simulink model "PMLSMDrive"  (R2024a)
settings: Solver=ode23t  StartTime=0.0  StopTime=10  RelTol=1e-3  AbsTol=1e-3  EnableMultiTasking=on
PreLoadFcn:
  | PMLSMDriveData;
values from neighbouring files (symbols this model uses):
  finalspeed = 0    [PMLSMDriveData.m]
  Fmax = 2000    [PMLSMDriveData.m]
  Ki_p = 100    [PMLSMDriveData.m]
  Ki_v = 250    [PMLSMDriveData.m]
  Kp_p = 200    [PMLSMDriveData.m]
  Kp_v = 250    [PMLSMDriveData.m]
  Ld = 0.01    [PMLSMDriveData.m]
  Lq = 0.01    [PMLSMDriveData.m]
  Np = pi/pitch    (= 31.4159265359)    [PMLSMDriveData.m]
  PM = 0.65    [PMLSMDriveData.m]
  Ts = 5e-5    (= 5e-05)    [PMLSMDriveData.m]
  Tsc = 1e-3    (= 0.001)    [PMLSMDriveData.m]
libraries: nesl_utility x12, fl_lib x7, ee_lib x5, eeTransforms x2, slpidlib x2, simulink x2, eePmsmCurrentController x1, eePwmGeneratorTwoLevel x1, dspsnks4 x1
CloseFcn:
  | try,close(h1_PMLSMDrive),end
  | clear h1_PMLSMDrive
  | 
  | clear PM Ld Lq L0 Rs mass pitch Np
  | clear Ts fsw Tsc Kp_id Ki_id Kp_iq Ki_iq
  | clear Kp_v Ki_v Kp_p Ki_p
Description:
  | Three-Phase PMLSM Drive
settings Model: Creator=The MathWorks, Inc.  LastModifiedBy=bkpou
settings SolverCC: AutoScaleAbsTol=off  MaxConsecutiveMinStep=2  ZeroCrossAlgorithm=Adaptive  AlgebraicLoopSolver=TrustRegion  MaxZcPerStep=1
settings DataIOCC: LimitDataPoints=on  MaxDataPoints=690000  SaveFormat=Array  ReturnWorkspaceOutputs=off  SignalLoggingName=logsout_PMLSMDrive
settings OptimizationCC: ReuseModelBlockBuffer=off  LifeSpan=inf
settings DebuggingCC: MaxConsecutiveZCsMsg=none  IgnoredZcDiagnostic=none  UnconnectedInputMsg=warning  UnconnectedOutputMsg=warning  UnconnectedLineMsg=warning  AllowSymbolicDim=off  PregeneratedLibrarySubsystemCodeDiagnostic=none  SFUnexpectedBacktrackingDiag=warning  SFNoUnconditionalDefaultTransitionDiag=warning  SFExecutionAtInitializationDiag=none  ArithmeticOperatorsInVariantConditions=warning
settings HardwareCC: ProdBitPerPointer=32  ProdBitPerSizeT=32  ProdBitPerPtrDiffT=32  ProdLargestAtomicFloat=None  ProdIntDivRoundTo=Undefined  ProdEndianess=Unspecified  ProdWordSize=32  ProdHWDeviceType=32-bit Generic
settings ModelReferenceCC: EnableRefExpFcnMdlSchedulingChecks=on  PropagateSignalLabelsOutOfModel=off
settings SFSimCC: SimUseLocalCustomCode=off
settings RTWCC: RTWUseLocalCustomCode=off  GPUComputeCapability=3.5  DLArmComputeVersion=19.05
settings CodeAppCC: StateflowObjectComments=on
settings GRTTargetCC: TargetLangStandard=C89/C90 (ANSI)
settings ConfigComp: CovMetricSettings=dw  CovSaveCumulativeToWorkspaceVar=on  CovSaveSingleToWorkspaceVar=on  CovExternalEMLEnable=off  CovSFcnEnable=off
settings SimscapeCC: SimscapeLogType=all  SimscapeLogSimulationStatistics=on  SimscapeLogName=simlog_PMLSMDrive  SimscapeLogDataHistory=690000

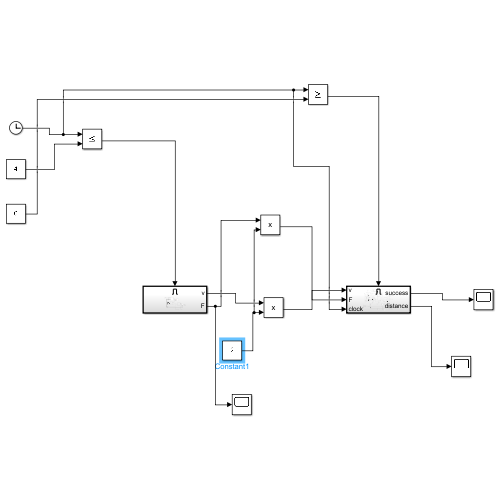
[thumbnail: Simulink's stored preview of the top-level diagram]
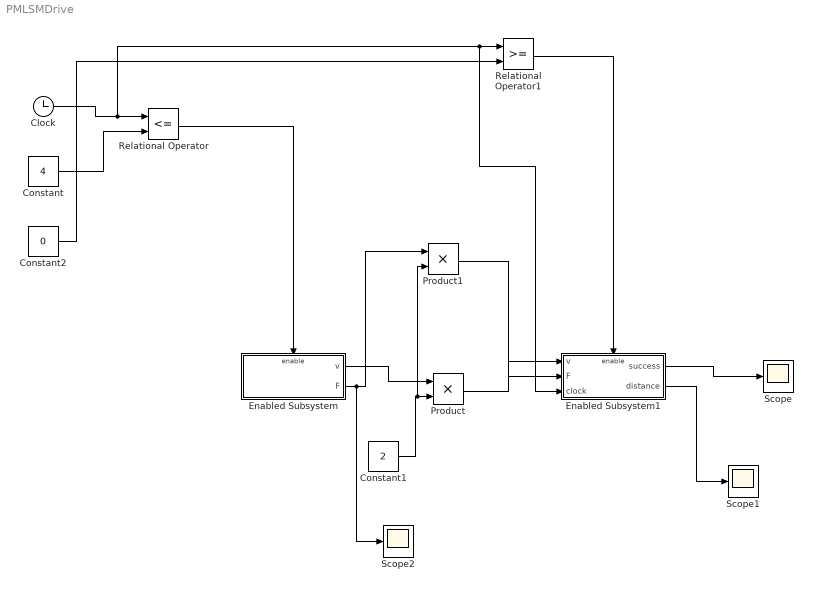
== system PMLSMDrive ==
  Clock : Clock
  Constant : Constant  Value=4
  Constant1 : Constant  Value=2
  Constant2 : Constant  Value=0
  Enabled Subsystem : Subsystem  TreatAsAtomicUnit=on
  Enabled Subsystem1 : Subsystem  TreatAsAtomicUnit=on
  Product : Product
  Product1 : Product
  Relational Operator : RelationalOperator  Operator=<=  OutDataTypeStr=boolean  RndMeth=Simplest  InputSameDT=off
  Relational Operator1 : RelationalOperator  OutDataTypeStr=boolean  RndMeth=Simplest  InputSameDT=off
  Scope : Scope
  Scope1 : Scope
  Scope2 : Scope
  wires:
  Clock/1 -> Enabled Subsystem1/3(clock), Relational Operator1/1, Relational Operator/1
  Constant/1 -> Relational Operator/2
  Relational Operator/1 -> Enabled Subsystem/Enable
  Relational Operator1/1 -> Enabled Subsystem1/Enable
  Enabled Subsystem/1(v) -> Product/1
  Constant1/1 -> Product1/2, Product/2
  Product/1 -> Enabled Subsystem1/1(v)
  Enabled Subsystem1/1(success) -> Scope/1
  Enabled Subsystem1/2(distance) -> Scope1/1
  Enabled Subsystem/2(F) -> Scope2/1, Product1/1
  Product1/1 -> Enabled Subsystem1/2(F)
  Constant2/1 -> Relational Operator1/2

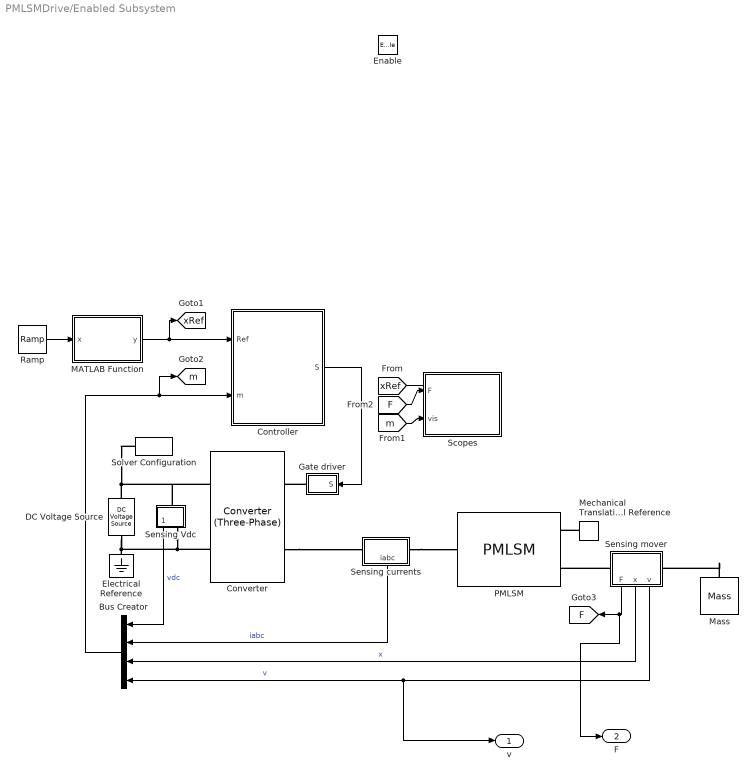
== system PMLSMDrive/Enabled Subsystem ==
  Enable : EnablePort
  Bus Creator : BusCreator  Inputs=4
  Controller : Subsystem
  Converter : ee_lib/Semiconductors & Converters/Converters/Converter (Three-Phase)  port_option=ee.enum.threePhasePort.composite  fidelity_option=ee.enum.converters.fidelity.detailed  device_type=ee.enum.converters.switchingdevice.igbt  K=0  Vf=0.8 V  Ron=0.001 Ohm  Rds=0.001 Ohm  Goff=1e-5 1/Ohm  Vgt=1 V  Vgt_off=-1 V  Ih=1 A  Vth=0.5 V  diode_param=ee.enum.converters.protectiondiode.nodynamics  diode_Vf=0.8 V  diode_Ron=0.001 Ohm  diode_Goff=1e-5 1/Ohm  diode_C=50 nF  diode_iRM=-235 A  diode_iF=300 A  diode_idot=-50 A/us  diode_trr_param=ee.enum.converters.diodetrr.trr_factor  diode_trr_factor=3  diode_trr=15 us  diode_Qrr=1.5e+3 s*uA  snubber_type=ee.enum.converters.snubber.exclude  Cs=1e-7 F  Rs=0.1 Ohm
  DC Voltage Source : ee_lib/Additional Components/SPICE Sources/DC Voltage Source  DC=220 V
  Electrical Reference : fl_lib/Electrical/Electrical Elements/Electrical Reference
  Gate driver : Subsystem
  MATLAB Function : MATLAB Function  TreatAsAtomicUnit=on
  Mass : fl_lib/Mechanical/Translational Elements/Mass  mass=mass kg  num_ports=foundation.enum.numPorts2.one  v_specify=off  v_priority=High  v=0 m/s  v_nominal_specify=off  v_nominal_value=1  v_nominal_unit=m/s  f_specify=off  f_priority=None  f=0 N  f_nominal_specify=off  f_nominal_value=1  f_nominal_unit=N
  Mechanical Translational Reference : fl_lib/Mechanical/Translational Elements/Mechanical Translational Reference
  PMLSM : ee_lib/Electromechanical/Permanent Magnet/PMLSM  port_option=ee.enum.threePhasePort.composite  winding_type=ee.enum.statorconnection.wye  machine_param=ee.enum.pmsm.parameterization.constant  polarPitch=pitch m  pmflux_param=ee.enum.pmfluxlin.fluxlinkage  pm_flux_linkage=PM Wb  force_constant=0.18 N/A  back_emf_constant=0.18 s*V/m  stator_param=ee.enum.statorparam.LdLqL0  Ld=Ld H  Lq=Lq H  idVec=[-200, 0, 200] A  iqVec=[-200, 0, 200] A  LdMatrix=0.00019 * ones(3, 3) H  LqMatrix=0.00025 * ones(3, 3) H  PmMatrix=0.03 * ones(3, 3) Wb  kfMatrix=0.18 * ones(3, 3) N/A  keMatrix=0.18 * ones(3, 3) s*V/m  L0=L0 H  Ls=0.0002 H  Lm=-0.00002 H  Ms=0.00002 H  Rs=Rs Ohm  zero_sequence=ee.enum.park.zerosequence.exclude  axes_param=ee.enum.rotorangle.qaxis  M=0 kg  lam=0 N/(m/s)  i_d_specify=on  i_d_priority=High  i_d=0 A  i_d_nominal_specify=off  i_d_nominal_value=1  i_d_nominal_unit=A  i_q_specify=on  i_q_priority=High  i_q=0 A  i_q_nominal_specify=off  i_q_nominal_value=1  i_q_nominal_unit=A  force_specify=off  force_priority=None  force=0 N  force_nominal_specify=off  force_nominal_value=1  force_nominal_unit=N  linear_velocity_specify=off  linear_velocity_priority=High  linear_velocity=0 m/s  linear_velocity_nominal_specify=off  linear_velocity_nominal_value=1  linear_velocity_nominal_unit=m/s  linear_position_specify=off  linear_position_priority=High  linear_position=0 m  linear_position_nominal_specify=off  linear_position_nominal_value=1  linear_position_nominal_unit=m  Tmeas=298.15 K  alpha=3.93e-3 1/K  alpha_flux=-0.001 1/K  stator_thermal_mass=100 J/K  rotor_thermal_mass=200 J/K  temperatureA_specify=off  temperatureA_priority=High  temperatureA=25 degC  temperatureA_nominal_specify=off  temperatureA_nominal_value=1  temperatureA_nominal_unit=degC  temperatureB_specify=off  temperatureB_priority=High  temperatureB=25 degC  temperatureB_nominal_specify=off  temperatureB_nominal_value=1  temperatureB_nominal_unit=degC  temperatureC_specify=off  temperatureC_priority=High  temperatureC=25 degC  temperatureC_nominal_specify=off  temperatureC_nominal_value=1  temperatureC_nominal_unit=degC  temperatureR_specify=off  temperatureR_priority=High  temperatureR=25 degC  temperatureR_nominal_specify=off  temperatureR_nominal_value=1  temperatureR_nominal_unit=degC
      settings: InternalSimscapePortConfiguration="{\"Bottom\":[],\"Left\":[{\"id\":\"N\",\"label\":\"~\",\"type\":\"foundation.electrical.three_phase\"}],\"Right\":[{\"id\":\"R\",\"label\":\"R\",\"type\":\"foundation.mechanical.translational.translational\"},{\"id\":\"C\",\"label\":\"C\",\"type\":\"foundation.mechanical.translational.translational\"}],\"Top\":[]}"
  Ramp : simulink/Sources/Ramp  slope=5  start=0  InitialOutput=0
  Scopes : Subsystem
  Sensing Vdc : Subsystem
      mask Display: disp('vdc')
  Sensing currents : Subsystem
      settings: PortSchema="{\"entries\":[{\"content\":{\"sides\":[{\"content\":{\"connectorIds\":[\"LConn1\"]},\"type\":\"ConnectorPlacement.EquallySpacedRectSide\",\"uuid\":\"0c76379d-baff-4140-87e0-7680e80a3e64\"},{\"content\":{\"connectorIds\":[\"RConn1\"],\"side\":\"RIGHT\"},\"type\":\"ConnectorPlacement.EquallySpacedRectSide\",\"uuid\":\"435fa78d-19d1-48b9-8f1c-afd8cf746df8\"},{\"content\":{\"connectorIds\":[],\"side\":\"TOP\"},\"type\":\"ConnectorPlacement.EquallySpacedRectSide\",\"uuid\":\"64f7027d-3f1c-43c6-9f97-24bcd914447a\"},{\"content\":{\"connectorIds\":[\"Out1\"],\"side\":\"BOTTOM\"},\"type\":\"ConnectorPlacement.EquallySpacedRectSide\",\"uuid\":\"10c10308-e912-4df5-9465-b109ad6411e6\"}]},\"type\":\"ConnectorPlacement.EquallySpacedConnector\",\"uuid\":\"559fa4aa-2e9f-4f72-acfb-6b72122ee549\"}],\"packageUris\":[\"http://schema.mathworks.com/mf0/Connector/R2020b\"],\"version\":\"1.0\"}"
      mask Display: disp('iabc')
  "Sensing mover " : Subsystem
      settings: PortSchema="{\"entries\":[{\"content\":{\"sides\":[{\"content\":{\"connectorIds\":[\"LConn1\"]},\"type\":\"ConnectorPlacement.EquallySpacedRectSide\",\"uuid\":\"6dd62e1f-51ba-4aba-a162-82178346648e\"},{\"content\":{\"connectorIds\":[\"RConn1\"],\"side\":\"RIGHT\"},\"type\":\"ConnectorPlacement.EquallySpacedRectSide\",\"uuid\":\"d7237c3a-82f8-4015-b1be-086487fff7ab\"},{\"content\":{\"connectorIds\":[],\"side\":\"TOP\"},\"type\":\"ConnectorPlacement.EquallySpacedRectSide\",\"uuid\":\"056d6889-c837-4b54-b9b7-572481429841\"},{\"content\":{\"connectorIds\":[\"Out1\",\"Out2\",\"Out3\"],\"side\":\"BOTTOM\"},\"type\":\"ConnectorPlacement.EquallySpacedRectSide\",\"uuid\":\"c892334a-0cdf-49f0-9b4f-3c9e9a0dee4e\"}]},\"type\":\"ConnectorPlacement.EquallySpacedConnector\",\"uuid\":\"04d69959-dab1-4865-ab7f-ace877df7771\"}],\"packageUris\":[\"http://schema.mathworks.com/mf0/Connector/R2020b\"],\"version\":\"1.0\"}"
  Solver Configuration : nesl_utility/Solver Configuration  PhysicalDomain=network_engine_domain  SubClassName=solver  LeftPortType=input  RightPortType=generic  Tones=[]  Harmonics=[]  SimulateNoise=off  Profile=off  UseLocalSampling=off  EnableSwitchedLinearOptims=on  FrequencyDomain=off  UseCCode=off  RelTol=0.001  AbsTol=1e-06  MinStep=1e-09  ToWorkspace=off  RevertToSquareIcSolve=off  NumHomotopyIterations=100  PhasorMode=off  PhasorModeNumHarmonics=1  ConsistencySolver=NEWTON_FTOL  IndexReductionMethod=DerivativeReplacement  DoDC=off  ResidualTolerance=1e-9  ConsistencyTolSource=GLOBAL  ConsistencyAbsTol=0.001  ConsistencyRelTol=0.001  ConsistencyTolFactor=0.001  UseLocalSolver=on  LocalSolverChoice=NE_PARTITIONING_ADVANCER  ResolveIndetEquations=on  FunctionEvalNumThread=1  LocalSolverSampleTime=Ts  DoFixedCost=on  MaxNonlinIter=4  MaxModeIter=2  ComputeImpulses=off  ImpulseIterations=2  LinearAlgebra=auto  LinearAlgebraNumThread=0  EquationFormulation=NE_TIME_EF  DelaysMemoryBudget=1024  AutomaticFiltering=on  FilteringTimeConstant=0.001  PartitionStorageMethod=AS_NEEDED  PartitionMemoryBudget=1024  PartitionMethod=ROBUST  MultibodyUseLocalSolver=off  MultibodyLocalSolverChoice=ODE1  MultibodyLocalSolverSampleTime=0.001
  v : Outport
  F : Outport  Port=2
  tag scope: F=global, m=global, xRef=global
  wires:
  Ramp/1 -> MATLAB Function/1(x)
  "Sensing mover "/2(x) -> Bus Creator/3  "x"
  Sensing currents/1(iabc) -> Bus Creator/2  "iabc"
  "Sensing mover "/3(v) -> v/1, Bus Creator/4  "v"
  Bus Creator/1 -> [m], Controller/2(m)
  [m] -> Scopes/2(vis)
  Controller/1(S) -> Gate driver/1(S)
  "Sensing mover "/1(F) -> F/1, [F]
  [F] -> Scopes/1(F)
  [xRef] -> ?
  MATLAB Function/1(y) -> [xRef], Controller/1(Ref)
  Sensing Vdc/1(vdc) -> Bus Creator/1  "vdc"
  connections:
  Converter/RConn2 -- DC Voltage Source/RConn1 -- Electrical Reference/LConn1 -- Sensing Vdc/RConn1
  Solver Configuration/RConn1 -- DC Voltage Source/LConn1 -- Sensing Vdc/LConn1 -- Converter/RConn1
  Mass/LConn1 -- "Sensing mover "/RConn1
  Gate driver/RConn1 -- Converter/LConn1
  Sensing currents/RConn1 -- PMLSM/LConn1
  "Sensing mover "/LConn1 -- PMLSM/RConn1
  Converter/LConn2 -- Sensing currents/LConn1
  Mechanical Translational Reference/LConn1 -- PMLSM/RConn2

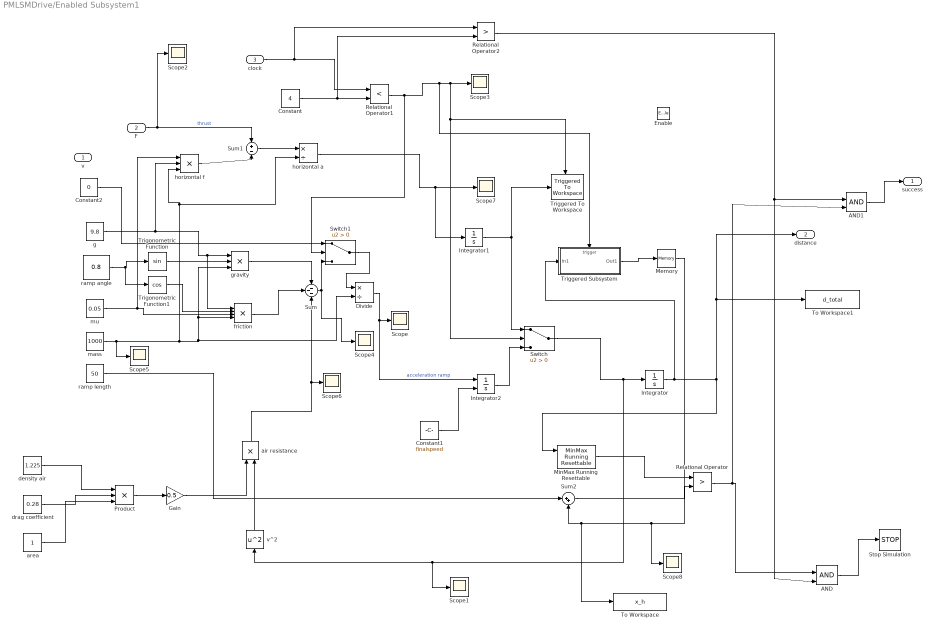
== system PMLSMDrive/Enabled Subsystem1 ==
  v : Inport
  F : Inport  Port=2
  clock : Inport  Port=3
  Enable : EnablePort
  AND : Logic  IconShape=distinctive  AllPortsSameDT=off  OutDataTypeStr=boolean
  AND1 : Logic  IconShape=distinctive  AllPortsSameDT=off  OutDataTypeStr=boolean
  Constant : Constant  Value=4
  Constant1 : Constant  Value=finalspeed
  Constant2 : Constant  Value=0
  Divide : Product  Inputs=*/
  Gain : Gain  Gain=0.5
  Integrator : Integrator
  Integrator1 : Integrator
  Integrator2 : Integrator  InitialConditionSource=external
  Memory : Memory
  MinMax Running Resettable : simulink/Math Operations/MinMax Running Resettable  Function=max  vinit=0.0
  Product : Product  Inputs=3
  Relational Operator : RelationalOperator  Operator=>  OutDataTypeStr=boolean  RndMeth=Simplest  InputSameDT=off
  Relational Operator1 : RelationalOperator  Operator=<  OutDataTypeStr=boolean  RndMeth=Simplest  InputSameDT=off
  Relational Operator2 : RelationalOperator  Operator=>  OutDataTypeStr=boolean  RndMeth=Simplest  InputSameDT=off
  Scope{,1..8} (9 alike) : Scope
  Stop Simulation : Stop
  Sum : Sum  Inputs=---
  Sum1 : Sum  Inputs=+-
  Sum2 : Sum  Inputs=|++
  Switch : Switch  Criteria=u2 > Threshold  SaturateOnIntegerOverflow=off  InputSameDT=off
  Switch1 : Switch  Criteria=u2 > Threshold  SaturateOnIntegerOverflow=off  InputSameDT=off
  To Workspace : ToWorkspace  VariableName=x_h  SaveFormat=Timeseries  SampleTime=-1
  To Workspace1 : ToWorkspace  VariableName=d_total  SaveFormat=Timeseries  SampleTime=-1
  Triggered Subsystem : Subsystem  TreatAsAtomicUnit=on
  Triggered To Workspace : dspsnks4/Triggered To Workspace  TriggerType=Falling edge  VariableName=finalspeed  Buffer=1  Save2DMode=2-D array (concatenate along first dimension)
      settings: FixptAsFi=off
  Trigonometric Function : Trigonometry
  Trigonometric Function1 : Trigonometry  Operator=cos
  air resistance : Product
  area : Constant
  density air : Constant  Value=1.225
  drag coefficient : Constant  Value=0.28
  friction : Product  Inputs=4
  g : Constant  Value=9.8
  gravity : Product  Inputs=3
  horizontal a : Product  Inputs=*/
  horizontal f : Product  Inputs=3
  mass : Constant  Value=1000
  mu : Constant  Value=0.05
  ramp angle : Constant  Value=0.8
  ramp length : Constant  Value=50
  v^2 : Math  Operator=square
  success : Outport
  distance : Outport  Port=2
  wires:
  ramp angle/1 -> Trigonometric Function1/1, Trigonometric Function/1
  mass/1 -> Scope5/1, horizontal a/2, horizontal f/3, Divide/2, friction/4, gravity/3
  g/1 -> horizontal f/2, friction/1, gravity/1
  Trigonometric Function/1 -> gravity/2
  Trigonometric Function1/1 -> friction/2
  mu/1 -> horizontal f/1, friction/3
  gravity/1 -> Sum/1
  friction/1 -> Sum/2
  Integrator/1 -> Triggered Subsystem/1(In1), MinMax Running Resettable/1, distance/1, To Workspace1/1
  MinMax Running Resettable/1 -> Relational Operator/1
  Relational Operator/1 -> AND1/2, AND/1
  density air/1 -> Product/1
  drag coefficient/1 -> Product/2
  area/1 -> Product/3
  Product/1 -> Gain/1
  Gain/1 -> air resistance/1
  air resistance/1 -> Scope6/1, Sum/3
  v^2/1 -> air resistance/2
  F/1 -> Sum1/1, Scope2/1  "thrust"
  horizontal f/1 -> Sum1/2
  Sum1/1 -> horizontal a/1
  horizontal a/1 -> Integrator1/1, Scope7/1
  Relational Operator1/1 -> Switch1/2, Triggered Subsystem/Trigger, Triggered To Workspace/Trigger, Switch/2, Scope3/1
  Integrator1/1 -> Switch/1, Triggered To Workspace/1
  Switch/1 -> Scope1/1, v^2/1, Integrator/1
  Integrator2/1 -> Switch/3
  Divide/1 -> Scope/1, Integrator2/1  "acceleration ramp"
  Switch1/1 -> Divide/1
  Constant2/1 -> Switch1/1
  Sum/1 -> Switch1/3, Scope4/1
  Constant/1 -> Relational Operator2/2, Relational Operator1/2
  clock/1 -> Relational Operator2/1, Relational Operator1/1
  Constant1/1 -> Integrator2/2
  ramp length/1 -> Sum2/1
  Sum2/1 -> Relational Operator/2
  Triggered Subsystem/1(Out1) -> Memory/1
  Memory/1 -> Scope8/1, To Workspace/1, Sum2/2
  Relational Operator2/1 -> AND1/1, AND/2
  AND/1 -> Stop Simulation/1
  AND1/1 -> success/1

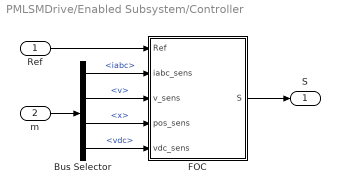
== system PMLSMDrive/Enabled Subsystem/Controller ==
  Ref : Inport
  m : Inport  Port=2
  Bus Selector : BusSelector  OutputSignals=iabc,v,x,vdc
  FOC : Subsystem
  S : Outport
  wires:
  Bus Selector/2 -> FOC/3(v_sens)  "<v>"
  Bus Selector/4 -> FOC/5(vdc_sens)  "<vdc>"
  Bus Selector/3 -> FOC/4(pos_sens)  "<x>"
  Bus Selector/1 -> FOC/2(iabc_sens)  "<iabc>"
  Ref/1 -> FOC/1(Ref)
  FOC/1(S) -> S/1
  m/1 -> Bus Selector/1

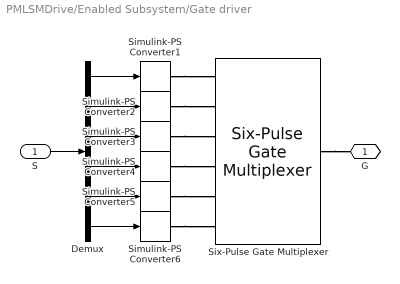
== system PMLSMDrive/Enabled Subsystem/Gate driver ==
  S : Inport
  Demux : Demux  Outputs=6
  Simulink-PS Converter{1..6} (6 alike) : nesl_utility/Simulink-PS Converter  PhysicalDomain=network_engine_domain  SubClassName=ps_input  LeftPortType=input  RightPortType=output  PseudoPeriodic=off  Frequencies=[]  NoiseDistribution=none  NoiseParameters=[]  Unit=1  AffineConversion=off  FilteringAndDerivatives=zero  SimscapeFilterOrder=1  InputFilterTimeConstant=0.001  UdotUserProvided=1
  Six-Pulse Gate Multiplexer : ee_lib/Semiconductors & Converters/Converters/Six-Pulse Gate Multiplexer  port_option=ee.enum.controlport.ps
  G : PMIOPort  Side=Right
  wires:
  Demux/1 -> Simulink-PS Converter1/1
  S/1 -> Demux/1
  Demux/4 -> Simulink-PS Converter4/1
  Demux/2 -> Simulink-PS Converter2/1
  Demux/3 -> Simulink-PS Converter3/1
  Demux/5 -> Simulink-PS Converter5/1
  Demux/6 -> Simulink-PS Converter6/1
  connections:
  Six-Pulse Gate Multiplexer/RConn1 -- G/RConn1
  Simulink-PS Converter1/RConn1 -- Six-Pulse Gate Multiplexer/LConn1
  Simulink-PS Converter3/RConn1 -- Six-Pulse Gate Multiplexer/LConn3
  Simulink-PS Converter5/RConn1 -- Six-Pulse Gate Multiplexer/LConn5
  Simulink-PS Converter6/RConn1 -- Six-Pulse Gate Multiplexer/LConn6
  Simulink-PS Converter4/RConn1 -- Six-Pulse Gate Multiplexer/LConn4
  Simulink-PS Converter2/RConn1 -- Six-Pulse Gate Multiplexer/LConn2

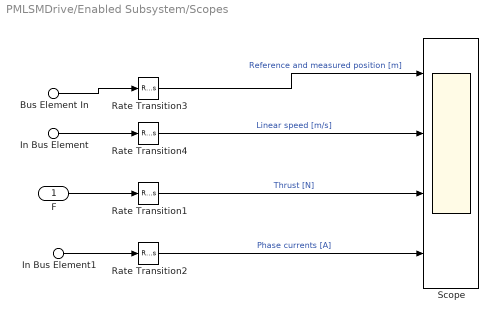
== system PMLSMDrive/Enabled Subsystem/Scopes ==
  F : Inport
  Bus Element In : Inport  Port=2  PortName=vis  Element=x
  In Bus Element : Inport  Port=2  PortName=vis  Element=v
  In Bus Element1 : Inport  Port=2  PortName=vis  Element=iabc
  Rate Transition{1..4} (4 alike) : RateTransition  OutPortSampleTime=Tsc
  Scope : Scope  NumInputPorts=4
  wires:
  In Bus Element/1 -> Rate Transition4/1
  Rate Transition2/1 -> Scope/4  "Phase currents [A]"
  In Bus Element1/1 -> Rate Transition2/1
  F/1 -> Rate Transition1/1
  Rate Transition1/1 -> Scope/3  "Thrust [N]"
  Bus Element In/1 -> Rate Transition3/1
  Rate Transition3/1 -> Scope/1  "Reference and measured position [m]"
  Rate Transition4/1 -> Scope/2  "Linear speed [m/s]"

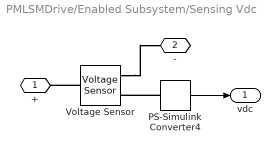
== system PMLSMDrive/Enabled Subsystem/Sensing Vdc ==
  PS-Simulink Converter4 : nesl_utility/PS-Simulink Converter  PhysicalDomain=network_engine_domain  SubClassName=ps_output  LeftPortType=input  RightPortType=output  PseudoPeriodic=off  Frequencies=[]  VectorFormat=1-D array  Unit=V  AffineConversion=off
  Voltage Sensor : fl_lib/Electrical/Electrical Sensors/Voltage Sensor
  + : PMIOPort  Side=Left
  - : PMIOPort  Port=2  Side=Right
  vdc : Outport
  wires:
  PS-Simulink Converter4/1 -> vdc/1
  connections:
  Voltage Sensor/LConn1 -- +/RConn1
  Voltage Sensor/RConn2 -- -/RConn1
  PS-Simulink Converter4/LConn1 -- Voltage Sensor/RConn1

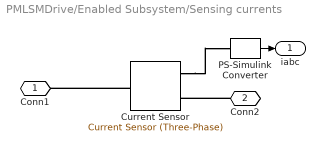
== system PMLSMDrive/Enabled Subsystem/Sensing currents ==
  Current Sensor : ee_lib/Sensors & Transducers/Current Sensor (Three-Phase)
  PS-Simulink Converter : nesl_utility/PS-Simulink Converter  PhysicalDomain=network_engine_domain  SubClassName=ps_output  LeftPortType=input  RightPortType=output  PseudoPeriodic=off  Frequencies=[]  VectorFormat=1-D array  Unit=A  AffineConversion=off
  Conn1 : PMIOPort  Side=Left
  Conn2 : PMIOPort  Port=2  Side=Right
  iabc : Outport
  wires:
  PS-Simulink Converter/1 -> iabc/1
  connections:
  Current Sensor/RConn1 -- PS-Simulink Converter/LConn1
  Conn2/RConn1 -- Current Sensor/RConn2
  Current Sensor/LConn1 -- Conn1/RConn1

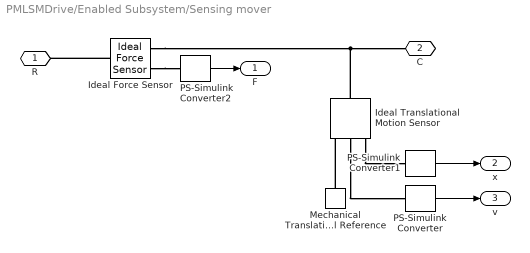
== system PMLSMDrive/Enabled Subsystem/Sensing mover  ==
  Ideal Force Sensor : fl_lib/Mechanical/Mechanical Sensors/Ideal Force Sensor
  Ideal Translational Motion Sensor : fl_lib/Mechanical/Mechanical Sensors/Ideal Translational Motion Sensor  reference=foundation.enum.MeasurementReference.difference  acceleration_port=false  velocity_port=true  position_port=true  offset=0 m
  Mechanical Translational Reference : fl_lib/Mechanical/Translational Elements/Mechanical Translational Reference
  PS-Simulink Converter : nesl_utility/PS-Simulink Converter  PhysicalDomain=network_engine_domain  SubClassName=ps_output  LeftPortType=input  RightPortType=output  PseudoPeriodic=off  Frequencies=[]  VectorFormat=1-D array  Unit=m/s  AffineConversion=off
  PS-Simulink Converter1 : nesl_utility/PS-Simulink Converter  PhysicalDomain=network_engine_domain  SubClassName=ps_output  LeftPortType=input  RightPortType=output  PseudoPeriodic=off  Frequencies=[]  VectorFormat=1-D array  Unit=m  AffineConversion=off
  PS-Simulink Converter2 : nesl_utility/PS-Simulink Converter  PhysicalDomain=network_engine_domain  SubClassName=ps_output  LeftPortType=input  RightPortType=output  PseudoPeriodic=off  Frequencies=[]  VectorFormat=1-D array  Unit=N  AffineConversion=off
  R : PMIOPort  Side=Left
  C : PMIOPort  Port=2  Side=Right
  F : Outport
  x : Outport  Port=2
  v : Outport  Port=3
  wires:
  PS-Simulink Converter2/1 -> F/1
  PS-Simulink Converter/1 -> v/1
  PS-Simulink Converter1/1 -> x/1
  connections:
  Ideal Force Sensor/LConn1 -- R/RConn1
  Ideal Force Sensor/RConn2 -- PS-Simulink Converter2/LConn1
  Ideal Force Sensor/RConn1 -- Ideal Translational Motion Sensor/LConn1 -- C/RConn1
  Ideal Translational Motion Sensor/RConn3 -- PS-Simulink Converter1/LConn1
  Ideal Translational Motion Sensor/RConn2 -- PS-Simulink Converter/LConn1
  Mechanical Translational Reference/LConn1 -- Ideal Translational Motion Sensor/RConn1

== system PMLSMDrive/Enabled Subsystem1/Triggered Subsystem ==
  In1 : Inport
  Trigger : TriggerPort  TriggerType=falling  VariantControl=(inherit)
  Out1 : Outport
  wires:
  In1/1 -> Out1/1

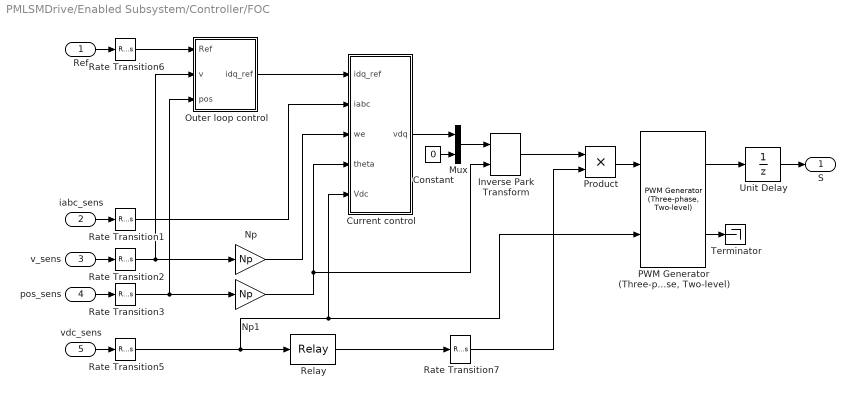
== system PMLSMDrive/Enabled Subsystem/Controller/FOC ==
  Ref : Inport
  iabc_sens : Inport  Port=2
  v_sens : Inport  Port=3
  pos_sens : Inport  Port=4
  vdc_sens : Inport  Port=5
  Constant : Constant  Value=0  SampleTime=-1
  Current control : Subsystem
  Inverse Park Transform : eeTransforms/Inverse Park Transform  AxisAlignment=Q-axis  PowerInvariant=off
  Mux : Mux  Inputs=2
  Np : Gain  Gain=Np
  Np1 : Gain  Gain=Np
  Outer loop control : Subsystem
  "PWM Generator (Three-phase, Two-level)" : eePwmGeneratorTwoLevel/PWM Generator (Three-phase, Two-level)  PWMMode=Continuous PWM (CPWM)  CPWMMode=SVM: space vector modulation  DPWMMode=60 DPWM: 60 degree discontinuous PWM  fsw=fsw  Ts=Ts
  Product : Product
  Rate Transition{1..3,5..6} (5 alike) : RateTransition  OutPortSampleTime=Tsc
  Rate Transition7 : RateTransition  OutPortSampleTime=Ts
  Relay : Relay  OnSwitchValue=24  OffSwitchValue=12
  Terminator : Terminator
  Unit Delay : UnitDelay  SampleTime=Ts  HasFrameUpgradeWarning=on
  S : Outport  VectorParamsAs1DForOutWhenUnconnected=off
  wires:
  v_sens/1 -> Rate Transition2/1
  pos_sens/1 -> Rate Transition3/1
  Current control/1(vdq) -> Mux/1
  Mux/1 -> Inverse Park Transform/1
  Rate Transition1/1 -> Current control/2(iabc)
  Outer loop control/1(idq_ref) -> Current control/1(idq_ref)
  Rate Transition5/1 -> Relay/1, "PWM Generator (Three-phase, Two-level)"/2, Current control/5(Vdc)
  vdc_sens/1 -> Rate Transition5/1
  iabc_sens/1 -> Rate Transition1/1
  Rate Transition3/1 -> Np1/1, Outer loop control/3(pos)
  Constant/1 -> Mux/2
  Relay/1 -> Rate Transition7/1
  Rate Transition2/1 -> Np/1, Outer loop control/2(v)
  Ref/1 -> Rate Transition6/1
  "PWM Generator (Three-phase, Two-level)"/2 -> Terminator/1
  Unit Delay/1 -> S/1
  Np/1 -> Current control/3(we)
  Np1/1 -> Current control/4(theta), Inverse Park Transform/2
  Rate Transition6/1 -> Outer loop control/1(Ref)
  "PWM Generator (Three-phase, Two-level)"/1 -> Unit Delay/1
  Product/1 -> "PWM Generator (Three-phase, Two-level)"/1
  Inverse Park Transform/1 -> Product/1
  Rate Transition7/1 -> Product/2

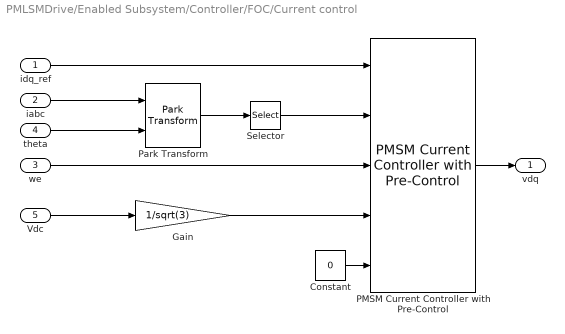
== system PMLSMDrive/Enabled Subsystem/Controller/FOC/Current control ==
  idq_ref : Inport
  iabc : Inport  Port=2
  we : Inport  Port=3
  theta : Inport  Port=4
  Vdc : Inport  Port=5
  Constant : Constant  Value=0  SampleTime=-1
  Gain : Gain  Gain=1/sqrt(3)
  PMSM Current Controller with Pre-Control : eePmsmCurrentController/PMSM Current Controller with Pre-Control  Kp_id=Kp_id  Ki_id=Ki_id  Kaw_id=1  Kp_iq=Kp_iq  Ki_iq=Ki_iq  Kaw_iq=1  Ts=-1  Tsd=Tsc  AxisPrio=Q-axis  ActZC=on  ActFF=on  idVect=[-200, 0, 200]  iqVect=[-200, 0, 200]  LdMatrix=Ld * ones(3, 3)  LqMatrix=Lq * ones(3, 3)  psimMatrix=PM * ones(3, 3)
  Park Transform : eeTransforms/Park Transform  AxisAlignment=Q-axis  PowerInvariant=off
  Selector : Selector  InputPortWidth=3  IndexOptions=Index vector (dialog)  Indices=[1 2]  OutputSizes=1
  vdq : Outport  VectorParamsAs1DForOutWhenUnconnected=off
  wires:
  Vdc/1 -> Gain/1
  iabc/1 -> Park Transform/1
  we/1 -> PMSM Current Controller with Pre-Control/3
  theta/1 -> Park Transform/2
  PMSM Current Controller with Pre-Control/1 -> vdq/1
  idq_ref/1 -> PMSM Current Controller with Pre-Control/1
  Constant/1 -> PMSM Current Controller with Pre-Control/5
  Selector/1 -> PMSM Current Controller with Pre-Control/2
  Gain/1 -> PMSM Current Controller with Pre-Control/4
  Park Transform/1 -> Selector/1

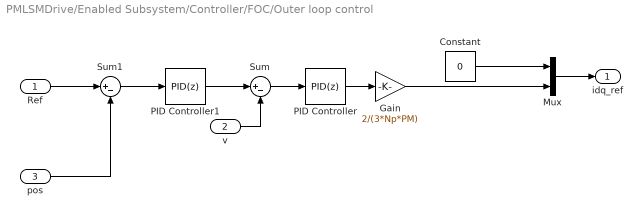
== system PMLSMDrive/Enabled Subsystem/Controller/FOC/Outer loop control ==
  Ref : Inport
  v : Inport  Port=2
  pos : Inport  Port=3
  Constant : Constant  Value=0
  Gain : Gain  Gain=2/(3*Np*PM)
  Mux : Mux  Inputs=2
  PID Controller : slpidlib/PID Controller  Controller=PID  Form=Parallel  TimeDomain=Discrete-time  UseExternalTs=off  SampleTime=Tsc  IntegratorMethod=Forward Euler  FilterMethod=Forward Euler  ControllerParametersSource=internal  P=Kp_v  I=Ki_v  UseKiTs=off  D=0  UseExternalDerivativeSource=off  N=100  UseFilter=on  TunerSelectOption=Transfer Function Based (PID Tuner App)  InitialConditionSource=internal  InitialConditionForIntegrator=0  InitialConditionForFilter=0  DifferentiatorICPrevScaledInput=0  ExternalReset=none  TrackingMode=off  Kt=1  LimitOutput=on  SatLimitsSource=internal  UpperSaturationLimit=Fmax*1.5  LowerSaturationLimit=-Fmax*1.5  LinearizeAsGain=on  AntiWindupMode=back-calculation  Kb=1000  LimitIntegrator=off  UpperIntegratorSaturationLimit=inf  LowerIntegratorSaturationLimit=-inf  POutMin=[]  POutMax=[]  IOutMin=[]  IOutMax=[]  DOutMin=[]  DOutMax=[]  NOutMin=[]  NOutMax=[]  SumOutMin=[]  SumOutMax=[]  SaturationOutMin=[]  SaturationOutMax=[]  PParamMin=[]  PParamMax=[]  IParamMin=[]  IParamMax=[]  DParamMin=[]  DParamMax=[]  NParamMin=[]  NParamMax=[]  KbParamMin=[]  KbParamMax=[]  KtParamMin=[]  KtParamMax=[]  KbOutMin=[]  KbOutMax=[]  KtOutMin=[]  KtOutMax=[]  IntegratorOutMin=[]  IntegratorOutMax=[]  FilterOutMin=[]  FilterOutMax=[]  SumI1OutMin=[]  SumI1OutMax=[]  SumI2OutMin=[]  SumI2OutMax=[]  SumI3OutMin=[]  SumI3OutMax=[]  SumI4OutMin=[]  SumI4OutMax=[]  SumDOutMin=[]  SumDOutMax=[]  DifferentiatorOutMin=[]  DifferentiatorOutMax=[]  FilterDiffOutCoefMin=[]  FilterDiffOutCoefMax=[]  ReciprocalOutMin=[]  ReciprocalOutMax=[]  SumDenOutMin=[]  SumDenOutMax=[]  SumNumOutMin=[]  SumNumOutMax=[]  DivideOutMin=[]  DivideOutMax=[]  UdiffTsProdOutMin=[]  UdiffTsProdOutMax=[]  NTsProdOutMin=[]  NTsProdOutMax=[]  UintegralTsProdOutMin=[]  UintegralTsProdOutMax=[]  UngainTsProdOutMin=[]  UngainTsProdOutMax=[]  ClampingZeroOutDataTypeStr=Inherit: Inherit via back propagation  ClampingZeroOutMin=[]  ClampingZeroOutMax=[]  FilterDenConstantOutDataTypeStr=Inherit: Inherit via back propagation  FilterDenConstantOutMin=[]  FilterDenConstantOutMax=[]  PCopyOutDataTypeStr=Inherit: Inherit via back propagation  PCopyOutMin=[]  PCopyOutMax=[]  NCopyOutDataTypeStr=Inherit: Inherit via back propagation  NCopyOutMin=[]  NCopyOutMax=[]  IntegratorContinuousStateAttributes=''  IntegratorStateMustResolveToSignalObject=off  IntegratorRTWStateStorageClass=Auto  FilterContinuousStateAttributes=''  FilterStateMustResolveToSignalObject=off  FilterRTWStateStorageClass=Auto  ParallelPVariant=InternalParameters  IdealPVariant=Disabled  IVariant=InternalParameters  DVariant=InternalParameters  IntegratorVariant=Discrete  SatVariant=Enabled  AWVariant=BackCalculation  PCopyVariant=Disabled  TRVariant=Disabled  FdbkBlocksVariant=Forward  IdealPFdbkVariant=Disabled  SatFdbkVariant=Disabled  DerivativeFilterVariant=ForwardEulerFilter  NVariant=InternalParameters  NCopyVariant=Disabled  FilterICVariant=InternalICsFilter  IntegratorICVariant=InternalICs  ExternalResetVariant=Disabled  TRSumVariant=Passthrough  SumFdbkVariant=Disabled  SumVariant=Sum_PID  TsampFilterVariant=InternalTs  TsampNgainVariant=Passthrough  TsampIntegralVariant=Disabled_SignalSpec  ExternalSaturationOutDataTypeStr=Inherit: Same as second input  DerivativeSourceVariant=ErrorSignal
  PID Controller1 : slpidlib/PID Controller  Controller=PID  Form=Parallel  TimeDomain=Discrete-time  UseExternalTs=off  SampleTime=Tsc  IntegratorMethod=Forward Euler  FilterMethod=Forward Euler  ControllerParametersSource=internal  P=Kp_p  I=Ki_p  UseKiTs=off  D=0  UseExternalDerivativeSource=off  N=100  UseFilter=on  TunerSelectOption=Transfer Function Based (PID Tuner App)  InitialConditionSource=internal  InitialConditionForIntegrator=0  InitialConditionForFilter=0  DifferentiatorICPrevScaledInput=0  ExternalReset=none  TrackingMode=off  Kt=1  LimitOutput=on  SatLimitsSource=internal  UpperSaturationLimit=10  LowerSaturationLimit=-10  LinearizeAsGain=on  AntiWindupMode=back-calculation  Kb=1000  LimitIntegrator=off  UpperIntegratorSaturationLimit=inf  LowerIntegratorSaturationLimit=-inf  POutMin=[]  POutMax=[]  IOutMin=[]  IOutMax=[]  DOutMin=[]  DOutMax=[]  NOutMin=[]  NOutMax=[]  SumOutMin=[]  SumOutMax=[]  SaturationOutMin=[]  SaturationOutMax=[]  PParamMin=[]  PParamMax=[]  IParamMin=[]  IParamMax=[]  DParamMin=[]  DParamMax=[]  NParamMin=[]  NParamMax=[]  KbParamMin=[]  KbParamMax=[]  KtParamMin=[]  KtParamMax=[]  KbOutMin=[]  KbOutMax=[]  KtOutMin=[]  KtOutMax=[]  IntegratorOutMin=[]  IntegratorOutMax=[]  FilterOutMin=[]  FilterOutMax=[]  SumI1OutMin=[]  SumI1OutMax=[]  SumI2OutMin=[]  SumI2OutMax=[]  SumI3OutMin=[]  SumI3OutMax=[]  SumI4OutMin=[]  SumI4OutMax=[]  SumDOutMin=[]  SumDOutMax=[]  DifferentiatorOutMin=[]  DifferentiatorOutMax=[]  FilterDiffOutCoefMin=[]  FilterDiffOutCoefMax=[]  ReciprocalOutMin=[]  ReciprocalOutMax=[]  SumDenOutMin=[]  SumDenOutMax=[]  SumNumOutMin=[]  SumNumOutMax=[]  DivideOutMin=[]  DivideOutMax=[]  UdiffTsProdOutMin=[]  UdiffTsProdOutMax=[]  NTsProdOutMin=[]  NTsProdOutMax=[]  UintegralTsProdOutMin=[]  UintegralTsProdOutMax=[]  UngainTsProdOutMin=[]  UngainTsProdOutMax=[]  ClampingZeroOutDataTypeStr=Inherit: Inherit via back propagation  ClampingZeroOutMin=[]  ClampingZeroOutMax=[]  FilterDenConstantOutDataTypeStr=Inherit: Inherit via back propagation  FilterDenConstantOutMin=[]  FilterDenConstantOutMax=[]  PCopyOutDataTypeStr=Inherit: Inherit via back propagation  PCopyOutMin=[]  PCopyOutMax=[]  NCopyOutDataTypeStr=Inherit: Inherit via back propagation  NCopyOutMin=[]  NCopyOutMax=[]  IntegratorContinuousStateAttributes=''  IntegratorStateMustResolveToSignalObject=off  IntegratorRTWStateStorageClass=Auto  FilterContinuousStateAttributes=''  FilterStateMustResolveToSignalObject=off  FilterRTWStateStorageClass=Auto  ParallelPVariant=InternalParameters  IdealPVariant=Disabled  IVariant=InternalParameters  DVariant=InternalParameters  IntegratorVariant=Discrete  SatVariant=Enabled  AWVariant=BackCalculation  PCopyVariant=Disabled  TRVariant=Disabled  FdbkBlocksVariant=Forward  IdealPFdbkVariant=Disabled  SatFdbkVariant=Disabled  DerivativeFilterVariant=ForwardEulerFilter  NVariant=InternalParameters  NCopyVariant=Disabled  FilterICVariant=InternalICsFilter  IntegratorICVariant=InternalICs  ExternalResetVariant=Disabled  TRSumVariant=Passthrough  SumFdbkVariant=Disabled  SumVariant=Sum_PID  TsampFilterVariant=InternalTs  TsampNgainVariant=Passthrough  TsampIntegralVariant=Disabled_SignalSpec  ExternalSaturationOutDataTypeStr=Inherit: Same as second input  DerivativeSourceVariant=ErrorSignal
  Sum : Sum  Inputs=|+-
  Sum1 : Sum  Inputs=|+-
  idq_ref : Outport  VectorParamsAs1DForOutWhenUnconnected=off
  wires:
  v/1 -> Sum/2
  Sum/1 -> PID Controller/1
  PID Controller/1 -> Gain/1
  Mux/1 -> idq_ref/1
  Constant/1 -> Mux/1
  PID Controller1/1 -> Sum/1
  Sum1/1 -> PID Controller1/1
  Ref/1 -> Sum1/1
  pos/1 -> Sum1/2
  Gain/1 -> Mux/2

== matlab function PMLSMDrive/Enabled Subsystem/MATLAB Function ==
  data: x input; y output
function y = exponential_function(x)
    A = 2; 
    B = 5;  
    y = A * exp(B * x);  % Exponential function
end
